simulink model "bo1808_foc_id0"  (R2024b)
settings: Solver=ode23tb  StartTime=0.0  StopTime=t_stop_foc  MaxStep=1e-5  RelTol=1e-3
model workspace (MAT data in the model file):
  B = 5.1285732711e-07
  Id_max = 0.6
  Iq_max = 0.6
  J = 1.4e-07
  Ki_id = 13571.6802635
  Ki_iq = 13571.6802635
  Ki_w = 0.279803284771
  Kp_id = 0.697433569097
  Kp_iq = 0.697433569097
  Kp_w = 0.0043730736291
  Ld = 0.00037
  Lq = 0.00037
  Rs = 7.2
  TL_nom = 0.0012
  TL_step_time = 0.04
  Vdc = 11.4
  Vdq_max = 6.58179306876
  pn = 4
  psi_f = 0.00106666666667
  speed_ref_rpm = 3000
  t_stop_foc = 0.1
  theta_e0 = 0
settings Model: Creator=26683  LastModifiedBy=26683

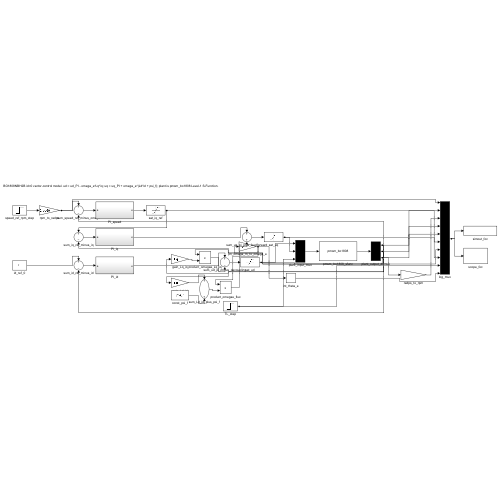
[thumbnail: Simulink's stored preview of the top-level diagram]
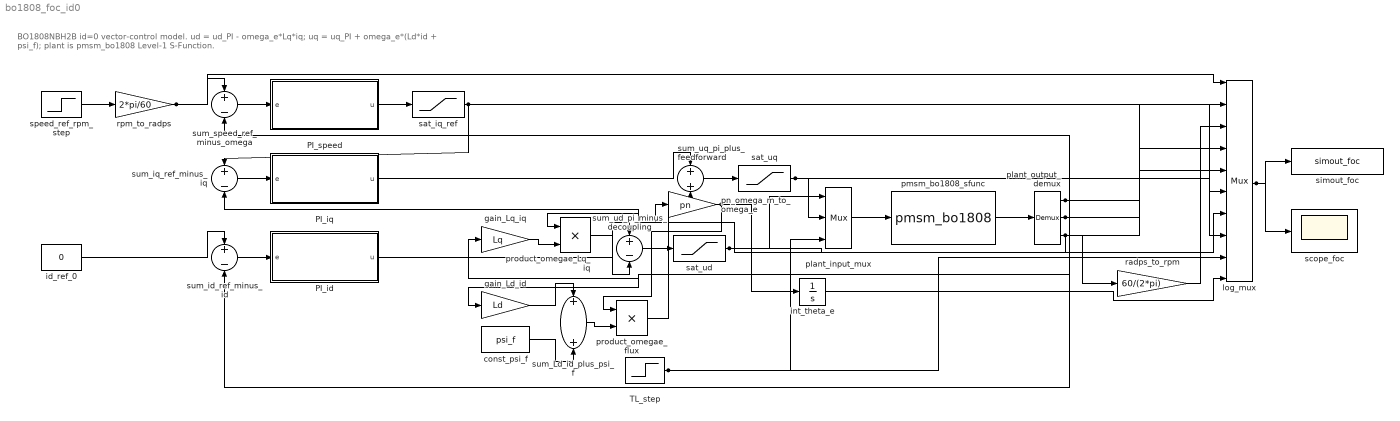
== system bo1808_foc_id0 ==
  note: BO1808NBH2B id=0 vector-control model. ud = ud_PI - omega_e*Lq*iq; uq = uq_PI + omega_e*(Ld*id + psi_f); plant is pmsm_bo1808 Level-1 S-Function.
  PI_id : Subsystem
  PI_iq : Subsystem
  PI_speed : Subsystem
  TL_step : Step  Time=TL_step_time  After=TL_nom  SampleTime=0
  const_psi_f : Constant  Value=psi_f
  gain_Ld_id : Gain  Gain=Ld
  gain_Lq_iq : Gain  Gain=Lq
  id_ref_0 : Constant  Value=0
  int_theta_e : Integrator  InitialCondition=theta_e0
  log_mux : Mux  Inputs=10
  plant_input_mux : Mux  Inputs=3
  plant_output_demux : Demux  Outputs=3
  pmsm_bo1808_sfunc : S-Function  FunctionName=pmsm_bo1808  SFunctionDeploymentMode=off  EnableBusSupport=off
  pn_omega_m_to_omega_e : Gain  Gain=pn
  product_omegae_Lq_iq : Product  Inputs=**
  product_omegae_flux : Product  Inputs=**
  radps_to_rpm : Gain  Gain=60/(2*pi)
  rpm_to_radps : Gain  Gain=2*pi/60
  sat_iq_ref : Saturate  UpperLimit=Iq_max  LowerLimit=-Iq_max
  sat_ud : Saturate  UpperLimit=Vdq_max  LowerLimit=-Vdq_max
  sat_uq : Saturate  UpperLimit=Vdq_max  LowerLimit=-Vdq_max
  scope_foc : Scope
  simout_foc : ToWorkspace  VariableName=simout_foc  SaveFormat=Structure With Time  SampleTime=-1
  speed_ref_rpm_step : Step  Time=0.005  After=speed_ref_rpm  SampleTime=0
  sum_Ld_id_plus_psi_f : Sum
  sum_id_ref_minus_id : Sum  Inputs=+-
  sum_iq_ref_minus_iq : Sum  Inputs=+-
  sum_speed_ref_minus_omega : Sum  Inputs=+-
  sum_ud_pi_minus_decoupling : Sum  Inputs=+-
  sum_uq_pi_plus_feedforward : Sum
  wires:
  speed_ref_rpm_step/1 -> rpm_to_radps/1
  rpm_to_radps/1 -> sum_speed_ref_minus_omega/1, log_mux/1
  sum_speed_ref_minus_omega/1 -> PI_speed/1(e)
  PI_speed/1(u) -> sat_iq_ref/1
  id_ref_0/1 -> sum_id_ref_minus_id/1
  sat_iq_ref/1 -> sum_iq_ref_minus_iq/1, log_mux/6
  sum_id_ref_minus_id/1 -> PI_id/1(e)
  sum_iq_ref_minus_iq/1 -> PI_iq/1(e)
  PI_id/1(u) -> sum_ud_pi_minus_decoupling/1
  product_omegae_Lq_iq/1 -> sum_ud_pi_minus_decoupling/2
  sum_ud_pi_minus_decoupling/1 -> sat_ud/1
  PI_iq/1(u) -> sum_uq_pi_plus_feedforward/1
  product_omegae_flux/1 -> sum_uq_pi_plus_feedforward/2
  sum_uq_pi_plus_feedforward/1 -> sat_uq/1
  sat_ud/1 -> plant_input_mux/1, log_mux/7
  sat_uq/1 -> plant_input_mux/2, log_mux/8
  TL_step/1 -> plant_input_mux/3, log_mux/9
  plant_input_mux/1 -> pmsm_bo1808_sfunc/1
  pmsm_bo1808_sfunc/1 -> plant_output_demux/1
  plant_output_demux/1 -> sum_id_ref_minus_id/2, gain_Ld_id/1, log_mux/4
  plant_output_demux/2 -> sum_iq_ref_minus_iq/2, gain_Lq_iq/1, log_mux/5
  plant_output_demux/3 -> sum_speed_ref_minus_omega/2, pn_omega_m_to_omega_e/1, radps_to_rpm/1, log_mux/2
  pn_omega_m_to_omega_e/1 -> product_omegae_Lq_iq/1, product_omegae_flux/1, int_theta_e/1
  gain_Lq_iq/1 -> product_omegae_Lq_iq/2
  gain_Ld_id/1 -> sum_Ld_id_plus_psi_f/1
  const_psi_f/1 -> sum_Ld_id_plus_psi_f/2
  sum_Ld_id_plus_psi_f/1 -> product_omegae_flux/2
  radps_to_rpm/1 -> log_mux/3
  int_theta_e/1 -> log_mux/10
  log_mux/1 -> simout_foc/1, scope_foc/1

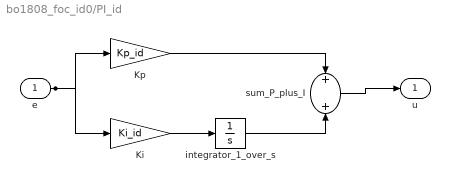
== system bo1808_foc_id0/PI_id ==
  e : Inport
  Ki : Gain  Gain=Ki_id
  Kp : Gain  Gain=Kp_id
  integrator_1_over_s : Integrator
  sum_P_plus_I : Sum
  u : Outport
  wires:
  e/1 -> Kp/1, Ki/1
  Kp/1 -> sum_P_plus_I/1
  Ki/1 -> integrator_1_over_s/1
  integrator_1_over_s/1 -> sum_P_plus_I/2
  sum_P_plus_I/1 -> u/1

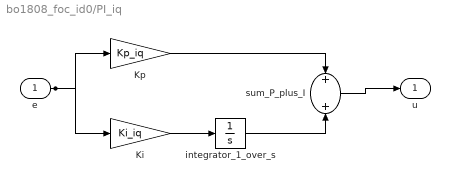
== system bo1808_foc_id0/PI_iq ==
  e : Inport
  Ki : Gain  Gain=Ki_iq
  Kp : Gain  Gain=Kp_iq
  integrator_1_over_s : Integrator
  sum_P_plus_I : Sum
  u : Outport
  wires:
  e/1 -> Kp/1, Ki/1
  Kp/1 -> sum_P_plus_I/1
  Ki/1 -> integrator_1_over_s/1
  integrator_1_over_s/1 -> sum_P_plus_I/2
  sum_P_plus_I/1 -> u/1

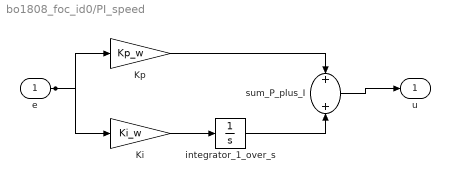
== system bo1808_foc_id0/PI_speed ==
  e : Inport
  Ki : Gain  Gain=Ki_w
  Kp : Gain  Gain=Kp_w
  integrator_1_over_s : Integrator
  sum_P_plus_I : Sum
  u : Outport
  wires:
  e/1 -> Kp/1, Ki/1
  Kp/1 -> sum_P_plus_I/1
  Ki/1 -> integrator_1_over_s/1
  integrator_1_over_s/1 -> sum_P_plus_I/2
  sum_P_plus_I/1 -> u/1
